simulink model "task_H_rea_mod"  (R2018a)
settings: Solver=ode4  StartTime=0.0  StopTime=10.0  FixedStep=0.01  RelTol=1e-3  EnableMultiTasking=on
values from neighbouring files (symbols this model uses):
  a0 = 1    [task_B_scr.m]    (also in task_E_scr.m = 0.5; task_H_real_scr.m = 0.5; task_H_scr.m = 0.5; task_J_scr.m = 0.5)
  b0 = 2    [task_B_scr.m]    (also in task_C_scr.m; task_D_scr.m; task_E_scr.m = 1; task_G_scr.m)
  nois_i = 1    [task_A_scr.m]    (also in task_B_scr.m; task_C_scr.m; task_D_scr.m; task_E_scr.m)
  nois_o = 1; sim('Task_A_mod',20)    [task_A_scr.m]    (also in task_B_scr.m = 1; sim('Task_B_mod',20); task_C_scr.m = 1; sim('Task_C_mod',2); task_D_scr.m = 1; sim('Task_D_mod',20); task_E_scr.m = 1; sim('Task_E_mod',20))
settings Model: Creator=Yurii  LastModifiedBy=Master
settings DataIOCC: LimitDataPoints=on  SaveFormat=Array
settings OptimizationCC: LifeSpan=inf
settings DebuggingCC: UnderspecifiedInitializationDetection=Classic  MergeDetectMultiDrivingBlocksExec=none  SolverPrmCheckMsg=warning  SFUnexpectedBacktrackingDiag=warning  SFNoUnconditionalDefaultTransitionDiag=warning  SFExecutionAtInitializationDiag=none
settings HardwareCC: ProdBitPerPointer=32  ProdBitPerSizeT=32  ProdBitPerPtrDiffT=32  ProdLargestAtomicFloat=None  ProdIntDivRoundTo=Undefined  ProdEndianess=Unspecified  ProdWordSize=32  ProdHWDeviceType=32-bit Generic
settings ModelReferenceCC: PropagateSignalLabelsOutOfModel=off
settings CodeAppCC: StateflowObjectComments=on
settings GRTTargetCC: TargetLangStandard=C89/C90 (ANSI)  GeneratePreprocessorConditionals=Disable all
settings ConfigComp: CovMetricSettings=dw  CovHtmlReporting=on  CovSaveCumulativeToWorkspaceVar=on  CovSaveSingleToWorkspaceVar=on  CovExternalEMLEnable=off

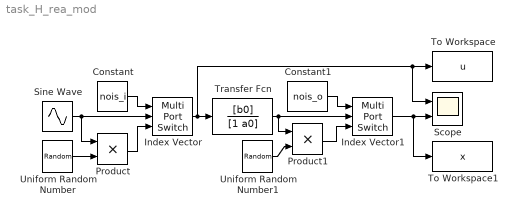
== system task_H_rea_mod ==
  Constant : Constant  Value=nois_i
  Constant1 : Constant  Value=nois_o
  Index Vector : MultiPortSwitch  DataPortOrder=Zero-based contiguous  Inputs=2  zeroidx=on
  Index Vector1 : MultiPortSwitch  DataPortOrder=Zero-based contiguous  Inputs=2  zeroidx=on
  Product : Product
  Product1 : Product
  Scope : Scope  NumInputPorts=2
  Sine Wave : Sin  SampleTime=0
  To Workspace : ToWorkspace  VariableName=u  SaveFormat=Timeseries  SampleTime=-1
  To Workspace1 : ToWorkspace  VariableName=x  SaveFormat=Timeseries  SampleTime=-1
  Transfer Fcn : TransferFcn  Numerator=[b0]  Denominator=[1 a0]
  Uniform Random Number : UniformRandomNumber  Minimum=0.9  Maximum=1.1  SampleTime=0
  Uniform Random Number1 : UniformRandomNumber  Minimum=0.9  Maximum=1.1  SampleTime=0
  wires:
  Sine Wave/1 -> Product/1, Index Vector/2
  Product/1 -> Index Vector/3
  Uniform Random Number/1 -> Product/2
  Constant/1 -> Index Vector/1
  Index Vector/1 -> Transfer Fcn/1, To Workspace/1, Scope/1
  Transfer Fcn/1 -> Index Vector1/2, Product1/1
  Product1/1 -> Index Vector1/3
  Uniform Random Number1/1 -> Product1/2
  Constant1/1 -> Index Vector1/1
  Index Vector1/1 -> To Workspace1/1, Scope/2
